simulink model "ARMAX_ZADANIE_1_2"  (Simulink 8.7)
settings: Solver=FixedStepDiscrete  StartTime=0.0  StopTime=Tend  RelTol=1e-3
values from neighbouring files (symbols this model uses):
  c1o = 0.99    [ZADANIE_1_2.m]    (also in ZADANIE_2_1.m = 0; Zad_1_1.m = 0; Zad_1_1_8_kolorowe.m; Zad_2_1_zapominanie.m = 0)
  fu = 0.025    [ZADANIE_1_2.m]    (also in ZADANIE_2_1.m)
  Td = 1500    [ZADANIE_1_2.m]    (also in ZADANIE_2_1.m = 500; Zad_1_1.m; Zad_1_1_8_kolorowe.m; Zad_2_1_zapominanie.m = 500)
  Tp = 0.1    [ZADANIE_1_2.m]    (also in ZADANIE_2_1.m; Zad_1_1.m; Zad_1_1_8_kolorowe.m; Zad_2_1_zapominanie.m)
libraries: simulink x2
settings Model: Creator=agnpi  LastModifiedBy=agnpi
settings DataIOCC: LimitDataPoints=off  SaveFormat=Dataset
settings DebuggingCC: UnderspecifiedInitializationDetection=Simplified  MergeDetectMultiDrivingBlocksExec=error
settings HardwareCC: ProdBitPerPointer=64  ProdLargestAtomicFloat=Float  ProdIntDivRoundTo=Zero  ProdEndianess=LittleEndian  ProdWordSize=64  ProdHWDeviceType=Intel->x86-64 (Windows64)
settings ModelReferenceCC: PropagateSignalLabelsOutOfModel=on
settings ConfigComp: CovModelRefEnable=off

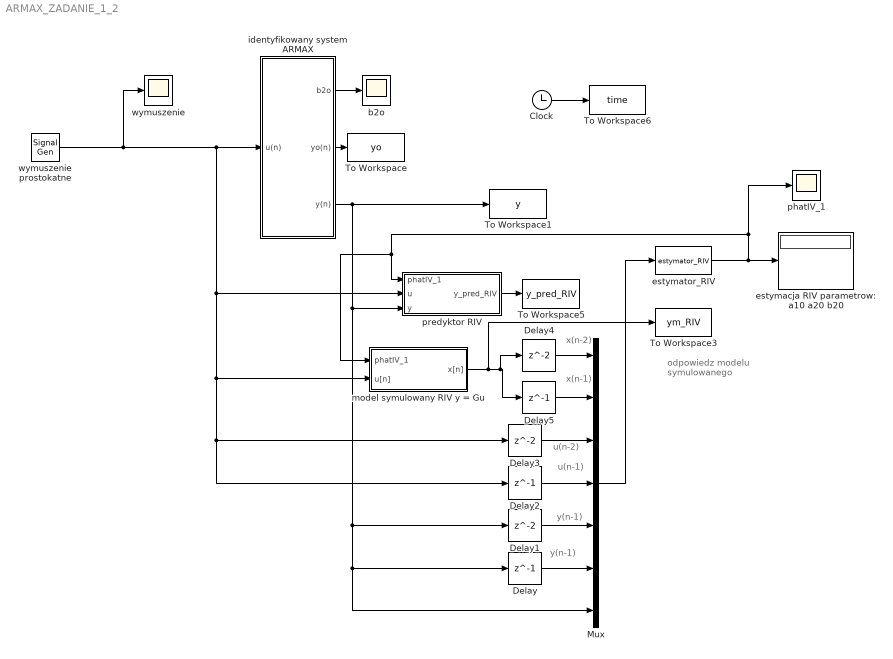
== system ARMAX_ZADANIE_1_2 ==
  note: odpowiedz modelu
      | symulowanego
  note: x(n-2)
  note: x(n-1)
  note: u(n-2)
  note: u(n-1)
  note: y(n-1)
  note: y(n-1)
  Clock : Clock
  Delay : Delay  DelayLength=1  InitialCondition=0
  Delay1 : Delay
  Delay2 : Delay  DelayLength=1  InitialCondition=0
  Delay3 : Delay
  Delay4 : Delay
  Delay5 : Delay  DelayLength=1  InitialCondition=0
  Mux : Mux  Inputs=7
  To Workspace : ToWorkspace  VariableName=yo  SampleTime=Tp
  To Workspace1 : ToWorkspace  VariableName=y  SampleTime=Tp
  To Workspace3 : ToWorkspace  VariableName=ym_RIV  SampleTime=Tp
  To Workspace5 : ToWorkspace  VariableName=y_pred_RIV  SampleTime=Tp
  To Workspace6 : ToWorkspace  VariableName=time  SampleTime=Tp
  b2o : Scope
  estymacja RIV parametrow: a10 a20 b20 : Display
  estymator_RIV : MATLABFcn  MATLABFcn=estymator_RIV  SampleTime=Tp
  identyfikowany system ARMAX : Subsystem
  model symulowany RIV y = Gu : Subsystem  SystemSampleTime=Tp
  phatIV_1 : Scope
  predyktor RIV : Subsystem
  wymuszenie : Scope
  wymuszenie prostokatne : SignalGenerator  WaveForm=square  Frequency=fu
  wires:
  wymuszenie prostokatne/1 -> wymuszenie/1, predyktor RIV/2(u), model symulowany RIV y = Gu/2(u[n]), Delay2/1, Delay3/1, identyfikowany system ARMAX/1(u(n))
  identyfikowany system ARMAX/1(b2o) -> b2o/1
  identyfikowany system ARMAX/2(yo(n)) -> To Workspace/1
  identyfikowany system ARMAX/3(y(n)) -> predyktor RIV/3(y), Mux/7, Delay/1, Delay1/1, To Workspace1/1
  Delay/1 -> Mux/6
  Delay1/1 -> Mux/5
  Delay2/1 -> Mux/4
  Delay3/1 -> Mux/3
  Delay4/1 -> Mux/1
  Delay5/1 -> Mux/2
  model symulowany RIV y = Gu/1(x[n]) -> To Workspace3/1, Delay4/1, Delay5/1
  Mux/1 -> estymator_RIV/1
  estymator_RIV/1 -> model symulowany RIV y = Gu/1(phatIV_1), predyktor RIV/1(phatIV_1), phatIV_1/1, estymacja RIV parametrow: a10 a20 b20/1
  predyktor RIV/1(y_pred_RIV) -> To Workspace5/1
  Clock/1 -> To Workspace6/1

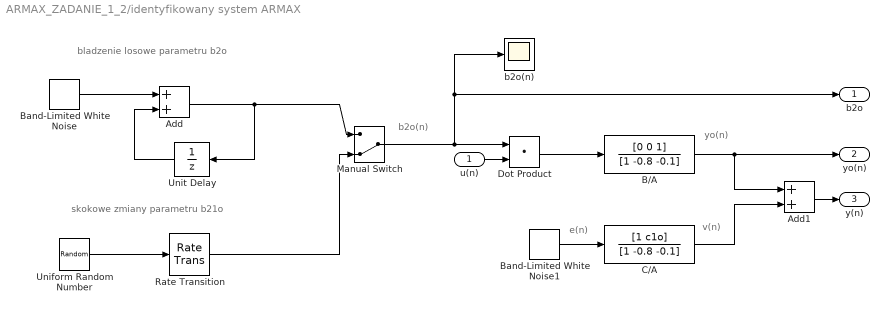
== system ARMAX_ZADANIE_1_2/identyfikowany system ARMAX ==
  note: e(n)
  note: v(n)
  note: yo(n)
  note: b2o(n)
  note: skokowe zmiany parametru b21o
  note: bladzenie losowe parametru b2o
  u(n) : Inport
  Add : Sum
  Add1 : Sum
  B/A : DiscreteFilter  Numerator=[0 0 1]  Denominator=[1 -0.8 -0.1]  SampleTime=Tp
  Band-Limited White Noise : simulink/Sources/Band-Limited White Noise  Cov=[0.00001*Tp]  Ts=Tp  seed=[23341]
  Band-Limited White Noise1 : simulink/Sources/Band-Limited White Noise  Cov=[0.001*Tp]  Ts=Tp  seed=[23341]
  C/A : DiscreteFilter  Numerator=[1 c1o]  Denominator=[1 -0.8 -0.1]  SampleTime=Tp
  Dot Product : DotProduct  InputSameDT=on  OutDataTypeStr=Inherit: Inherit via internal rule
  Manual Switch : ManualSwitch  CurrentSetting=0
  Rate Transition : RateTransition  X0=0.5  OutPortSampleTime=Tp
  Uniform Random Number : UniformRandomNumber  Minimum=0.1  Maximum=0.8  Seed=2  SampleTime=Td
  Unit Delay : UnitDelay  SampleTime=Tp
  b2o(n) : Scope
  b2o : Outport
  yo(n) : Outport  Port=2
  y(n) : Outport  Port=3
  wires:
  Band-Limited White Noise/1 -> Add/1
  Add/1 -> Unit Delay/1, Manual Switch/1
  Unit Delay/1 -> Add/2
  Uniform Random Number/1 -> Rate Transition/1
  Rate Transition/1 -> Manual Switch/2
  Manual Switch/1 -> Dot Product/1, b2o/1, b2o(n)/1
  Dot Product/1 -> B/A/1
  C/A/1 -> Add1/2
  B/A/1 -> Add1/1, yo(n)/1
  Band-Limited White Noise1/1 -> C/A/1
  u(n)/1 -> Dot Product/2
  Add1/1 -> y(n)/1

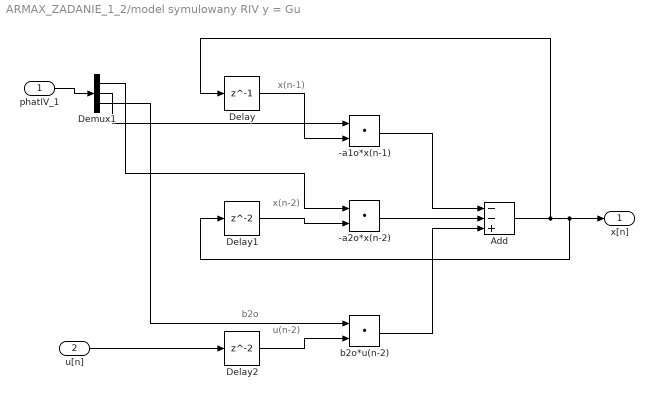
== system ARMAX_ZADANIE_1_2/model symulowany RIV y = Gu ==
  note: x(n-1)
  note: x(n-2)
  note: u(n-2)
  note: b2o
  phatIV_1 : Inport
  u[n] : Inport  Port=2
  -a1o*x(n-1) : DotProduct  InputSameDT=on  OutDataTypeStr=Inherit: Inherit via internal rule
  -a2o*x(n-2) : DotProduct  InputSameDT=on  OutDataTypeStr=Inherit: Inherit via internal rule
  Add : Sum  Inputs=--+
  Delay : Delay  DelayLength=1  InitialCondition=0  SampleTime=Tp
  Delay1 : Delay  InitialCondition=0  SampleTime=Tp
  Delay2 : Delay  InitialCondition=0  SampleTime=Tp
  Demux1 : Demux  Outputs=3
  b2o*u(n-2) : DotProduct  InputSameDT=on  OutDataTypeStr=Inherit: Inherit via internal rule
  x[n] : Outport
  wires:
  -a1o*x(n-1)/1 -> Add/1
  -a2o*x(n-2)/1 -> Add/2
  b2o*u(n-2)/1 -> Add/3
  u[n]/1 -> Delay2/1
  Add/1 -> Delay/1, Delay1/1, x[n]/1
  phatIV_1/1 -> Demux1/1
  Demux1/3 -> b2o*u(n-2)/1
  Delay2/1 -> b2o*u(n-2)/2
  Delay1/1 -> -a2o*x(n-2)/2
  Delay/1 -> -a1o*x(n-1)/2
  Demux1/1 -> -a2o*x(n-2)/1
  Demux1/2 -> -a1o*x(n-1)/1

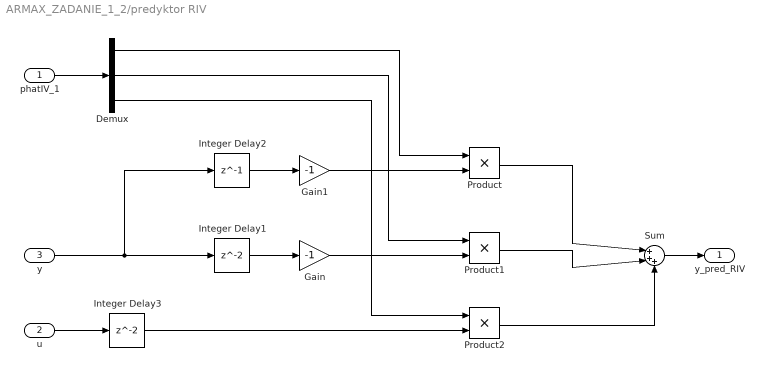
== system ARMAX_ZADANIE_1_2/predyktor RIV ==
  phatIV_1 : Inport
  u : Inport  Port=2
  y : Inport  Port=3
  Demux : Demux  Outputs=3
  Gain : Gain  Gain=-1
  Gain1 : Gain  Gain=-1
  Integer Delay1 : Delay  InputProcessing=Inherited  SampleTime=Tp
  Integer Delay2 : Delay  DelayLength=1  InputProcessing=Inherited  SampleTime=Tp
  Integer Delay3 : Delay  InputProcessing=Inherited  SampleTime=Tp
  Product : Product
  Product1 : Product
  Product2 : Product
  Sum : Sum  Inputs=|+++
  y_pred_RIV : Outport
  wires:
  u/1 -> Integer Delay3/1
  y/1 -> Integer Delay2/1, Integer Delay1/1
  Integer Delay1/1 -> Gain/1
  Integer Delay2/1 -> Gain1/1
  phatIV_1/1 -> Demux/1
  Sum/1 -> y_pred_RIV/1
  Product2/1 -> Sum/3
  Product1/1 -> Sum/2
  Product/1 -> Sum/1
  Gain1/1 -> Product/2
  Gain/1 -> Product1/2
  Integer Delay3/1 -> Product2/2
  Demux/1 -> Product/1
  Demux/2 -> Product1/1
  Demux/3 -> Product2/1
